simulink model "Circuit"  (R2020b)
settings: Solver=VariableStepAuto  StartTime=0.0  StopTime=10.0  RelTol=1e-3
settings Model: Creator=smart  LastModifiedBy=smart

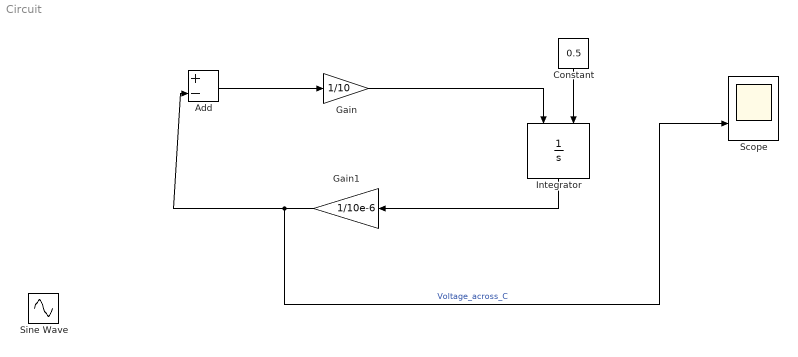
== system Circuit ==
  Add : Sum  Inputs=+-
  Constant : Constant  Value=0.5
  Gain : Gain  Gain=1/10
  Gain1 : Gain  Gain=1/10e-6
  Integrator : Integrator  InitialConditionSource=external
  Scope : Scope  NumInputPorts=2
  Sine Wave : Sin  SampleTime=0
  wires:
  ? -> Scope/1, Add/1  "input_voltage"
  Add/1 -> Gain/1
  Gain/1 -> Integrator/1
  Integrator/1 -> Gain1/1
  Gain1/1 -> Scope/2, Add/2  "Voltage_across_C"
  Constant/1 -> Integrator/2
